simulink model "common_3"  (R2015b)
settings: Solver=ode4  StartTime=0.0  StopTime=tmax  FixedStep=0.001  RelTol=1e-3
undefined symbols (not defined in the file): dq1_init, dq2_init, g, ki, kp, l, l10, l20, para, q1_init, q2_init
settings Model: Creator=Administrator  LastModifiedBy=Administrator

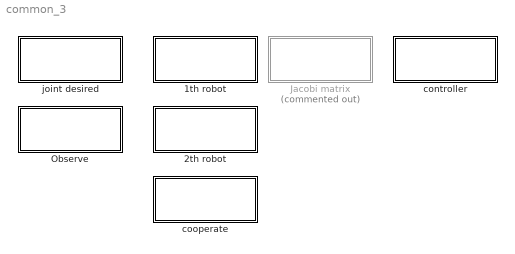
== system common_3 ==
  1th robot : Subsystem
  2th robot : Subsystem
  Jacobi matrix : Subsystem  Commented=on
  Observe : Subsystem
  controller : Subsystem
  cooperate : Subsystem
  joint desired : Subsystem

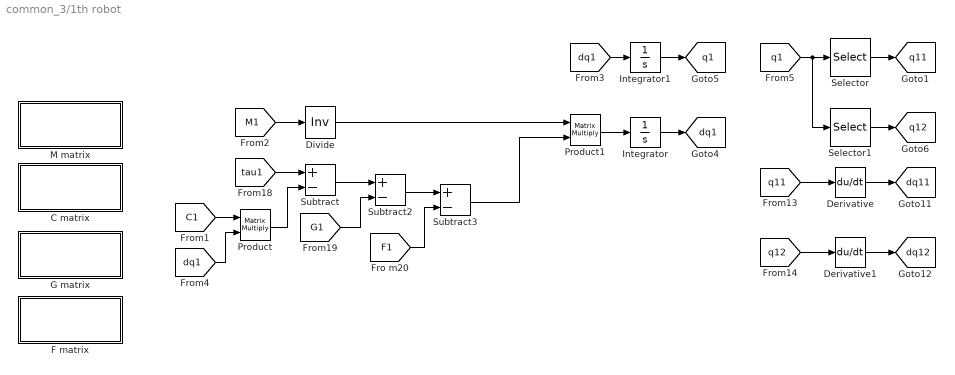
== system common_3/1th robot ==
  C matrix : Subsystem
  Derivative : Derivative
  "Derivative1 " : Derivative
  Divide : Product  Inputs=/  Multiplication=Matrix(*)
  F matrix : Subsystem
  G matrix : Subsystem
  Integrator : Integrator  InitialCondition=dq1_init
  Integrator1 : Integrator  InitialCondition=q1_init
  M matrix : Subsystem
  Product : Product  Multiplication=Matrix(*)
  Product1 : Product  Multiplication=Matrix(*)
  Selector : Selector  InputPortWidth=2  IndexOptions=Index vector (dialog)  Indices=[1]  OutputSizes=1
  Selector1 : Selector  InputPortWidth=2  IndexOptions=Index vector (dialog)  Indices=[2]  OutputSizes=1
  Subtract : Sum  Inputs=+-
  Subtract2 : Sum  Inputs=+-
  Subtract3 : Sum  Inputs=+-
  tag scope: dq11=global, dq12=global, dq1=global, q11=global, q12=global, q1=global
  wires:
  Integrator/1 -> [dq1]
  [dq1] -> Integrator1/1
  Integrator1/1 -> [q1]
  Selector/1 -> [q11]
  Selector1/1 -> [q12]
  [q1] -> Selector/1, Selector1/1
  [q11] -> Derivative/1
  Derivative/1 -> [dq11]
  [q12] -> "Derivative1 "/1
  "Derivative1 "/1 -> [dq12]
  [M1] -> Divide/1
  Product1/1 -> Integrator/1
  Divide/1 -> Product1/1
  [tau1] -> Subtract/1
  [C1] -> Product/1
  Product/1 -> Subtract/2
  Subtract/1 -> Subtract2/1
  [G1] -> Subtract2/2
  Subtract2/1 -> Subtract3/1
  [F1] -> Subtract3/2
  Subtract3/1 -> Product1/2
  [dq1] -> Product/2

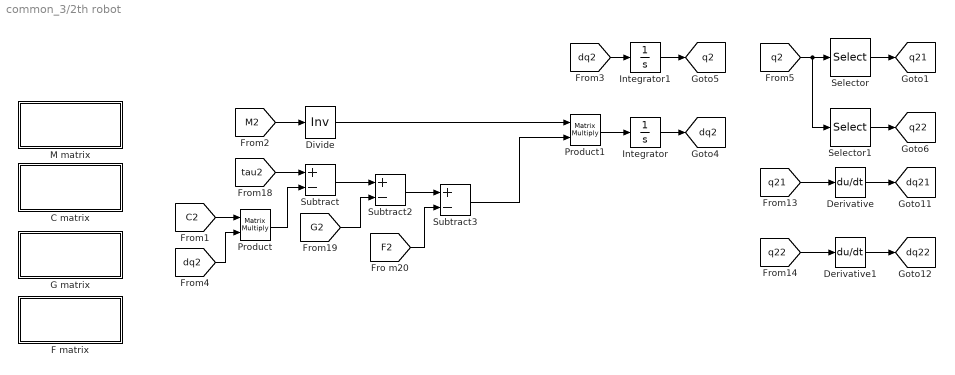
== system common_3/2th robot ==
  C matrix : Subsystem
  Derivative : Derivative
  "Derivative1 " : Derivative
  Divide : Product  Inputs=/  Multiplication=Matrix(*)
  F matrix : Subsystem
  G matrix : Subsystem
  Integrator : Integrator  InitialCondition=dq2_init
  Integrator1 : Integrator  InitialCondition=q2_init
  M matrix : Subsystem
  Product : Product  Multiplication=Matrix(*)
  Product1 : Product  Multiplication=Matrix(*)
  Selector : Selector  InputPortWidth=2  IndexOptions=Index vector (dialog)  Indices=[1]  OutputSizes=1
  Selector1 : Selector  InputPortWidth=2  IndexOptions=Index vector (dialog)  Indices=[2]  OutputSizes=1
  Subtract : Sum  Inputs=+-
  Subtract2 : Sum  Inputs=+-
  Subtract3 : Sum  Inputs=+-
  tag scope: dq21=global, dq22=global, dq2=global, q21=global, q22=global, q2=global
  wires:
  [dq2] -> Product/2
  Subtract3/1 -> Product1/2
  [F2] -> Subtract3/2
  Subtract2/1 -> Subtract3/1
  [G2] -> Subtract2/2
  Subtract/1 -> Subtract2/1
  Product/1 -> Subtract/2
  [C2] -> Product/1
  [tau2] -> Subtract/1
  Divide/1 -> Product1/1
  Product1/1 -> Integrator/1
  [M2] -> Divide/1
  "Derivative1 "/1 -> [dq22]
  [q22] -> "Derivative1 "/1
  Derivative/1 -> [dq21]
  [q21] -> Derivative/1
  [q2] -> Selector1/1, Selector/1
  Selector1/1 -> [q22]
  Selector/1 -> [q21]
  Integrator1/1 -> [q2]
  [dq2] -> Integrator1/1
  Integrator/1 -> [dq2]

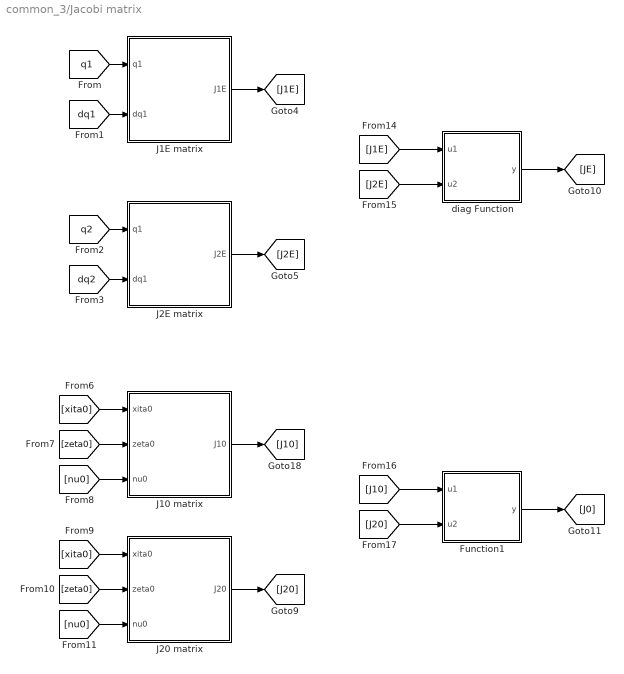
== system common_3/Jacobi matrix ==
  " Function1" : MATLAB Function  TreatAsAtomicUnit=on
  J10 matrix : Subsystem
  J1E matrix : Subsystem
  J20 matrix : Subsystem
  J2E matrix : Subsystem
  diag Function : MATLAB Function  TreatAsAtomicUnit=on
  wires:
  [q1] -> J1E matrix/1(q1)
  [dq1] -> J1E matrix/2(dq1)
  [q2] -> J2E matrix/1(q1)
  [dq2] -> J2E matrix/2(dq1)
  J1E matrix/1(J1E) -> [J1E]
  J2E matrix/1(J2E) -> [J2E]
  [xita0] -> J10 matrix/1(xita0)
  [xita0] -> J20 matrix/1(xita0)
  [zeta0] -> J20 matrix/2(zeta0)
  [nu0] -> J20 matrix/3(nu0)
  [zeta0] -> J10 matrix/2(zeta0)
  [nu0] -> J10 matrix/3(nu0)
  J10 matrix/1(J10) -> [J10]
  J20 matrix/1(J20) -> [J20]
  [J1E] -> diag Function/1(u1)
  [J2E] -> diag Function/2(u2)
  diag Function/1(y) -> [JE]
  [J10] -> " Function1"/1(u1)
  [J20] -> " Function1"/2(u2)
  " Function1"/1(y) -> [J0]

== system common_3/Observe ==
  Scope{,1..4} (5 alike) : Scope  NumInputPorts=4
  wires:
  [q11] -> Scope/1
  [q12] -> Scope/2
  [q21] -> Scope/3
  [q22] -> Scope/4
  [dq11] -> Scope1/1
  [dq12] -> Scope1/2
  [dq21] -> Scope1/3
  [dq22] -> Scope1/4
  [M1] -> Scope2/1
  [C1] -> Scope2/2
  [G1] -> Scope2/3
  [F1] -> Scope2/4
  [M2] -> Scope3/1
  [C2] -> Scope3/2
  [G2] -> Scope3/3
  [F2] -> Scope3/4
  [qd] -> Scope4/1
  [dqd] -> Scope4/2
  [q] -> Scope4/3
  [dq] -> Scope4/4

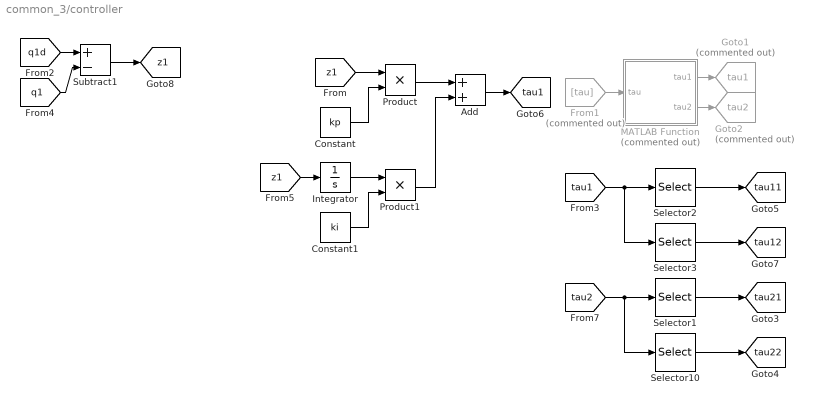
== system common_3/controller ==
  Add : Sum
  Constant : Constant  Value=kp
  Constant1 : Constant  Value=ki
  From1 : From  Commented=on  GotoTag=tau  TagVisibility=global
  Goto1 : Goto  Commented=on  GotoTag=tau1  TagVisibility=global
  Goto2 : Goto  Commented=on  GotoTag=tau2  TagVisibility=global
  Integrator : Integrator
  MATLAB Function : MATLAB Function  Commented=on  TreatAsAtomicUnit=on
  Product : Product
  Product1 : Product
  Selector1 : Selector  InputPortWidth=2  IndexOptions=Index vector (dialog)  Indices=[1]  OutputSizes=1
  Selector10 : Selector  InputPortWidth=2  IndexOptions=Index vector (dialog)  Indices=[2]  OutputSizes=1
  Selector2 : Selector  InputPortWidth=2  IndexOptions=Index vector (dialog)  Indices=[1]  OutputSizes=1
  Selector3 : Selector  InputPortWidth=2  IndexOptions=Index vector (dialog)  Indices=[2]  OutputSizes=1
  Subtract1 : Sum  Inputs=+-
  tag scope: tau11=global, tau12=global, tau1=global, tau21=global, tau22=global, z1=global
  wires:
  [z1] -> Product/1
  Constant/1 -> Product/2
  Product/1 -> Add/1
  Constant1/1 -> Product1/2
  Add/1 -> [tau1]
  From1/1 -> MATLAB Function/1(tau)
  MATLAB Function/1(tau1) -> Goto1/1
  MATLAB Function/2(tau2) -> Goto2/1
  Selector2/1 -> [tau11]
  Selector3/1 -> [tau12]
  [tau1] -> Selector3/1, Selector2/1
  Selector1/1 -> [tau21]
  Selector10/1 -> [tau22]
  [tau2] -> Selector1/1, Selector10/1
  [z1] -> Integrator/1
  Integrator/1 -> Product1/1
  Product1/1 -> Add/2
  [q1d] -> Subtract1/1
  [q1] -> Subtract1/2
  Subtract1/1 -> [z1]

== system common_3/cooperate ==
  MATLAB Function : MATLAB Function  TreatAsAtomicUnit=on
  Matrix Concatenate : Concatenate  Mode=Multidimensional array
  Matrix Concatenate1 : Concatenate  Mode=Multidimensional array
  tag scope: C=global, F=global, G=global, M=global, dq=global, q=global
  wires:
  [M1] -> MATLAB Function/1(M1)
  [M2] -> MATLAB Function/2(M2)
  [C1] -> MATLAB Function/3(C1)
  [C2] -> MATLAB Function/4(C2)
  MATLAB Function/1(M) -> [M]
  MATLAB Function/2(C) -> [C]
  [G1] -> MATLAB Function/5(G1)
  [G2] -> MATLAB Function/6(G2)
  MATLAB Function/3(G) -> [G]
  MATLAB Function/4(F) -> [F]
  [F1] -> MATLAB Function/7(F1)
  [F2] -> MATLAB Function/8(F2)
  [q1] -> Matrix Concatenate/1
  [q2] -> Matrix Concatenate/2
  Matrix Concatenate/1 -> [q]
  [dq1] -> Matrix Concatenate1/1
  [dq2] -> Matrix Concatenate1/2
  Matrix Concatenate1/1 -> [dq]

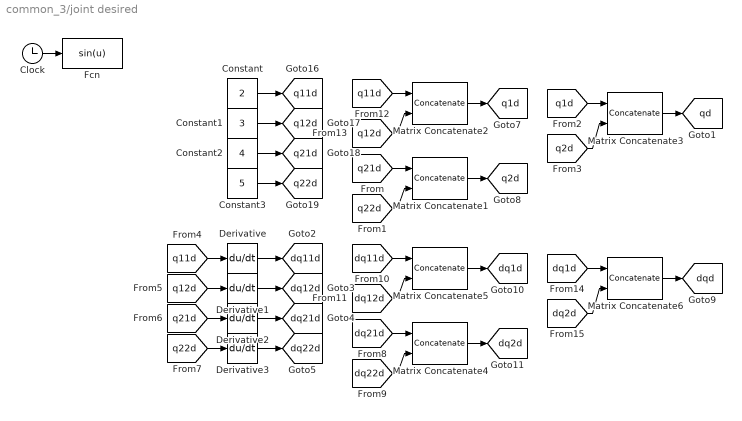
== system common_3/joint desired ==
  Clock : Clock
  Constant : Constant  Value=2
  Constant1 : Constant  Value=3
  Constant2 : Constant  Value=4
  Constant3 : Constant  Value=5
  Derivative{,1..3} (4 alike) : Derivative
  Fcn : Fcn  Expr=sin(u)
  Matrix Concatenate{1..6} (6 alike) : Concatenate  Mode=Multidimensional array
  tag scope: dq11d=global, dq12d=global, dq1d=global, dq21d=global, dq22d=global, dq2d=global, dqd=global, q11d=global, q12d=global, q1d=global, q21d=global, q22d=global, q2d=global, qd=global
  wires:
  Constant/1 -> [q11d]
  Constant3/1 -> [q22d]
  Constant2/1 -> [q21d]
  Constant1/1 -> [q12d]
  [q11d] -> Derivative/1
  Derivative/1 -> [dq11d]
  [q12d] -> Derivative1/1
  Derivative1/1 -> [dq12d]
  [q21d] -> Derivative2/1
  Derivative2/1 -> [dq21d]
  [q22d] -> Derivative3/1
  Derivative3/1 -> [dq22d]
  Matrix Concatenate3/1 -> [qd]
  Clock/1 -> Fcn/1
  [q11d] -> Matrix Concatenate2/1
  [q12d] -> Matrix Concatenate2/2
  Matrix Concatenate2/1 -> [q1d]
  [q21d] -> Matrix Concatenate1/1
  [q22d] -> Matrix Concatenate1/2
  Matrix Concatenate1/1 -> [q2d]
  [q1d] -> Matrix Concatenate3/1
  [q2d] -> Matrix Concatenate3/2
  Matrix Concatenate6/1 -> [dqd]
  [dq11d] -> Matrix Concatenate5/1
  [dq12d] -> Matrix Concatenate5/2
  Matrix Concatenate5/1 -> [dq1d]
  [dq21d] -> Matrix Concatenate4/1
  [dq22d] -> Matrix Concatenate4/2
  Matrix Concatenate4/1 -> [dq2d]
  [dq1d] -> Matrix Concatenate6/1
  [dq2d] -> Matrix Concatenate6/2

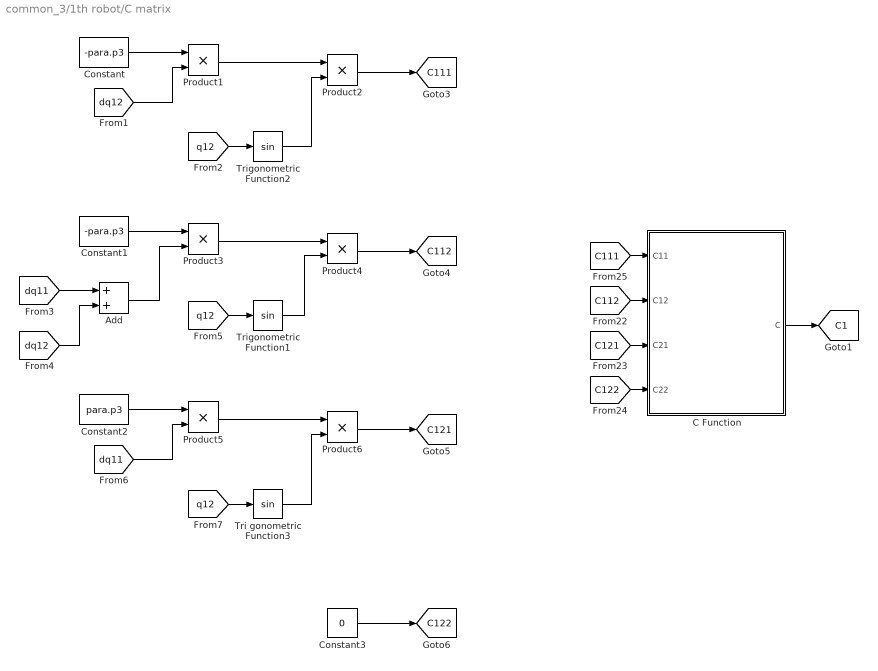
== system common_3/1th robot/C matrix ==
  Add : Sum
  C Function : MATLAB Function  TreatAsAtomicUnit=on
  Constant : Constant  Value=-para.p3
  Constant1 : Constant  Value=-para.p3
  Constant2 : Constant  Value=para.p3
  Constant3 : Constant  Value=0
  Product{1..6} (6 alike) : Product
  Tri gonometric Function3 : Trigonometry
  Trigonometric Function1 : Trigonometry
  Trigonometric Function2 : Trigonometry
  tag scope: C111=global, C112=global, C121=global, C122=global, C1=global
  wires:
  [C111] -> C Function/1(C11)
  [C112] -> C Function/2(C12)
  [C121] -> C Function/3(C21)
  [C122] -> C Function/4(C22)
  Constant/1 -> Product1/1
  [dq12] -> Product1/2
  Product1/1 -> Product2/1
  [q12] -> Trigonometric Function2/1
  Trigonometric Function2/1 -> Product2/2
  Product2/1 -> [C111]
  Constant1/1 -> Product3/1
  [dq11] -> Add/1
  [dq12] -> Add/2
  Add/1 -> Product3/2
  Product3/1 -> Product4/1
  [q12] -> Trigonometric Function1/1
  Trigonometric Function1/1 -> Product4/2
  Product4/1 -> [C112]
  Constant2/1 -> Product5/1
  [dq11] -> Product5/2
  Product5/1 -> Product6/1
  [q12] -> Tri gonometric Function3/1
  Tri gonometric Function3/1 -> Product6/2
  Product6/1 -> [C121]
  Constant3/1 -> [C122]
  C Function/1(C) -> [C1]

== system common_3/1th robot/F matrix ==
  Constant : Constant  Value=0.2
  Constant1 : Constant  Value=0.2
  F Function2 : MATLAB Function  TreatAsAtomicUnit=on
  Product : Product
  Product1 : Product
  Sign : Signum
  Sign1 : Signum
  tag scope: F11=global, F12=global, F1=global
  wires:
  F Function2/1(F) -> [F1]
  [F11] -> F Function2/1(F11)
  [F12] -> F Function2/2(F21)
  Constant/1 -> Product/1
  Sign/1 -> Product/2
  [dq11] -> Sign/1
  Product/1 -> [F11]
  Constant1/1 -> Product1/1
  Sign1/1 -> Product1/2
  [dq12] -> Sign1/1
  Product1/1 -> [F12]

== system common_3/1th robot/G matrix ==
  Constant : Constant  Value=para.p4*g
  Constant1 : Constant  Value=para.p5*g
  Constant2 : Constant  Value=para.p5*g
  G Function1 : MATLAB Function  TreatAsAtomicUnit=on
  Product1 : Product
  Product2 : Product
  Product3 : Product
  Subtract1 : Sum
  Subtract4 : Sum
  Subtract5 : Sum
  Trigonometric Function1 : Trigonometry  Operator=cos
  Trigonometric Function2 : Trigonometry  Operator=cos
  Trigonometric Function3 : Trigonometry  Operator=cos
  tag scope: G11=global, G12=global, G1=global
  wires:
  [G11] -> G Function1/1(G11)
  [G12] -> G Function1/2(G21)
  G Function1/1(G) -> [G1]
  Constant/1 -> Product1/1
  Trigonometric Function2/1 -> Product1/2
  [q11] -> Trigonometric Function2/1
  Product1/1 -> Subtract4/1
  Constant2/1 -> Product2/1
  Subtract5/1 -> Trigonometric Function3/1
  [q11] -> Subtract5/1
  [q12] -> Subtract5/2
  Trigonometric Function3/1 -> Product2/2
  Product2/1 -> Subtract4/2
  Subtract4/1 -> [G11]
  Constant1/1 -> Product3/1
  Subtract1/1 -> Trigonometric Function1/1
  [q11] -> Subtract1/1
  [q12] -> Subtract1/2
  Product3/1 -> [G12]
  Trigonometric Function1/1 -> Product3/2

== system common_3/1th robot/M matrix ==
  Constant1 : Constant  Value=2*para.p3
  Constant2 : Constant  Value=para.p1+para.p2
  Constant3 : Constant  Value=para.p2
  Constant4 : Constant  Value=para.p3
  Constant5 : Constant  Value=para.p2
  M Function1 : MATLAB Function  TreatAsAtomicUnit=on
  Product1 : Product
  Product2 : Product
  Subtract1 : Sum
  Subtract2 : Sum
  Trigonometric Function1 : Trigonometry  Operator=cos
  Trigonometric Function8 : Trigonometry  Operator=cos
  tag scope: M111=global, M112=global, M121=global, M122=global, M1=global
  wires:
  M Function1/1(M) -> [M1]
  [M111] -> M Function1/1(M11)
  [M112] -> M Function1/2(M12)
  [M121] -> M Function1/3(M21)
  [M122] -> M Function1/4(M22)
  [q12] -> Trigonometric Function8/1
  Constant2/1 -> Subtract1/1
  Constant1/1 -> Product1/1
  Trigonometric Function8/1 -> Product1/2
  Product1/1 -> Subtract1/2
  Subtract2/1 -> [M121], [M112]
  Constant5/1 -> [M122]
  Subtract1/1 -> [M111]
  Constant3/1 -> Subtract2/1
  Constant4/1 -> Product2/1
  [q12] -> Trigonometric Function1/1
  Trigonometric Function1/1 -> Product2/2
  Product2/1 -> Subtract2/2

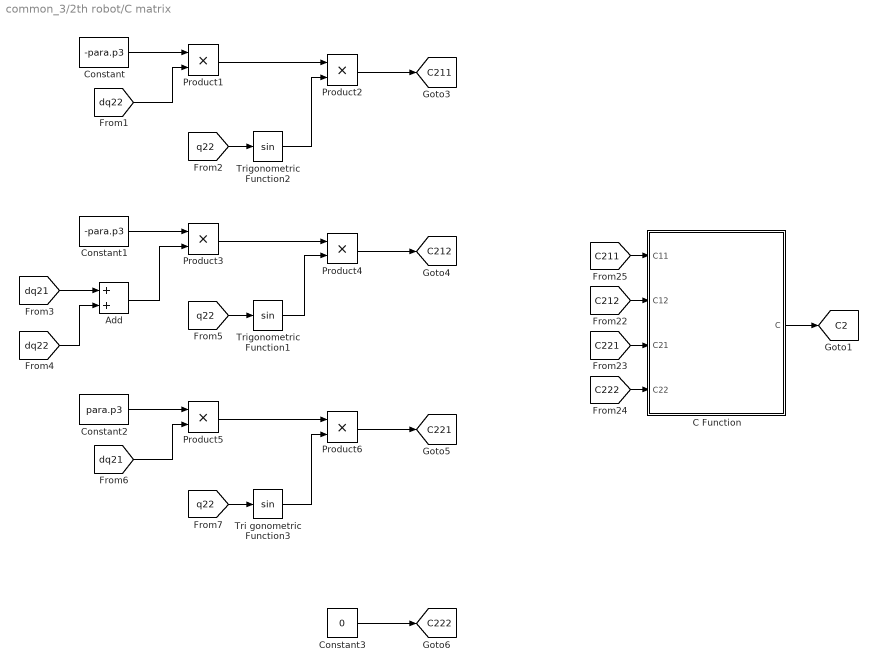
== system common_3/2th robot/C matrix ==
  Add : Sum
  C Function : MATLAB Function  TreatAsAtomicUnit=on
  Constant : Constant  Value=-para.p3
  Constant1 : Constant  Value=-para.p3
  Constant2 : Constant  Value=para.p3
  Constant3 : Constant  Value=0
  Product{1..6} (6 alike) : Product
  Tri gonometric Function3 : Trigonometry
  Trigonometric Function1 : Trigonometry
  Trigonometric Function2 : Trigonometry
  tag scope: C211=global, C212=global, C221=global, C222=global, C2=global
  wires:
  C Function/1(C) -> [C2]
  Constant3/1 -> [C222]
  Product6/1 -> [C221]
  Tri gonometric Function3/1 -> Product6/2
  [q22] -> Tri gonometric Function3/1
  Product5/1 -> Product6/1
  [dq21] -> Product5/2
  Constant2/1 -> Product5/1
  Product4/1 -> [C212]
  Trigonometric Function1/1 -> Product4/2
  [q22] -> Trigonometric Function1/1
  Product3/1 -> Product4/1
  Add/1 -> Product3/2
  [dq22] -> Add/2
  [dq21] -> Add/1
  Constant1/1 -> Product3/1
  Product2/1 -> [C211]
  Trigonometric Function2/1 -> Product2/2
  [q22] -> Trigonometric Function2/1
  Product1/1 -> Product2/1
  [dq22] -> Product1/2
  Constant/1 -> Product1/1
  [C222] -> C Function/4(C22)
  [C221] -> C Function/3(C21)
  [C212] -> C Function/2(C12)
  [C211] -> C Function/1(C11)

== system common_3/2th robot/F matrix ==
  Constant : Constant  Value=0.2
  Constant1 : Constant  Value=0.2
  F Function2 : MATLAB Function  TreatAsAtomicUnit=on
  Product : Product
  Product1 : Product
  Sign : Signum
  Sign1 : Signum
  tag scope: F21=global, F22=global, F2=global
  wires:
  Product1/1 -> [F22]
  [dq22] -> Sign1/1
  Sign1/1 -> Product1/2
  Constant1/1 -> Product1/1
  Product/1 -> [F21]
  [dq21] -> Sign/1
  Sign/1 -> Product/2
  Constant/1 -> Product/1
  [F22] -> F Function2/2(F21)
  [F21] -> F Function2/1(F11)
  F Function2/1(F) -> [F2]

== system common_3/2th robot/G matrix ==
  Constant : Constant  Value=para.p4*g
  Constant1 : Constant  Value=para.p5*g
  Constant2 : Constant  Value=para.p5*g
  G Function1 : MATLAB Function  TreatAsAtomicUnit=on
  Product1 : Product
  Product2 : Product
  Product3 : Product
  Subtract1 : Sum
  Subtract4 : Sum
  Subtract5 : Sum
  Trigonometric Function1 : Trigonometry  Operator=cos
  Trigonometric Function2 : Trigonometry  Operator=cos
  Trigonometric Function3 : Trigonometry  Operator=cos
  tag scope: G21=global, G22=global, G2=global
  wires:
  Trigonometric Function1/1 -> Product3/2
  Product3/1 -> [G22]
  [q22] -> Subtract1/2
  [q21] -> Subtract1/1
  Subtract1/1 -> Trigonometric Function1/1
  Constant1/1 -> Product3/1
  Subtract4/1 -> [G21]
  Product2/1 -> Subtract4/2
  Trigonometric Function3/1 -> Product2/2
  [q22] -> Subtract5/2
  [q21] -> Subtract5/1
  Subtract5/1 -> Trigonometric Function3/1
  Constant2/1 -> Product2/1
  Product1/1 -> Subtract4/1
  [q21] -> Trigonometric Function2/1
  Trigonometric Function2/1 -> Product1/2
  Constant/1 -> Product1/1
  G Function1/1(G) -> [G2]
  [G22] -> G Function1/2(G21)
  [G21] -> G Function1/1(G11)

== system common_3/2th robot/M matrix ==
  Constant1 : Constant  Value=2*para.p3
  Constant2 : Constant  Value=para.p1+para.p2
  Constant3 : Constant  Value=para.p2
  Constant4 : Constant  Value=para.p3
  Constant5 : Constant  Value=para.p2
  M Function1 : MATLAB Function  TreatAsAtomicUnit=on
  Product1 : Product
  Product2 : Product
  Subtract1 : Sum
  Subtract2 : Sum
  Trigonometric Function1 : Trigonometry  Operator=cos
  Trigonometric Function8 : Trigonometry  Operator=cos
  tag scope: M211=global, M212=global, M221=global, M222=global, M2=global
  wires:
  Product2/1 -> Subtract2/2
  Trigonometric Function1/1 -> Product2/2
  [q22] -> Trigonometric Function1/1
  Constant4/1 -> Product2/1
  Constant3/1 -> Subtract2/1
  Subtract1/1 -> [M211]
  Constant5/1 -> [M222]
  Subtract2/1 -> [M212], [M221]
  Product1/1 -> Subtract1/2
  Trigonometric Function8/1 -> Product1/2
  Constant1/1 -> Product1/1
  Constant2/1 -> Subtract1/1
  [q22] -> Trigonometric Function8/1
  [M222] -> M Function1/4(M22)
  [M221] -> M Function1/3(M21)
  [M212] -> M Function1/2(M12)
  [M211] -> M Function1/1(M11)
  M Function1/1(M) -> [M2]

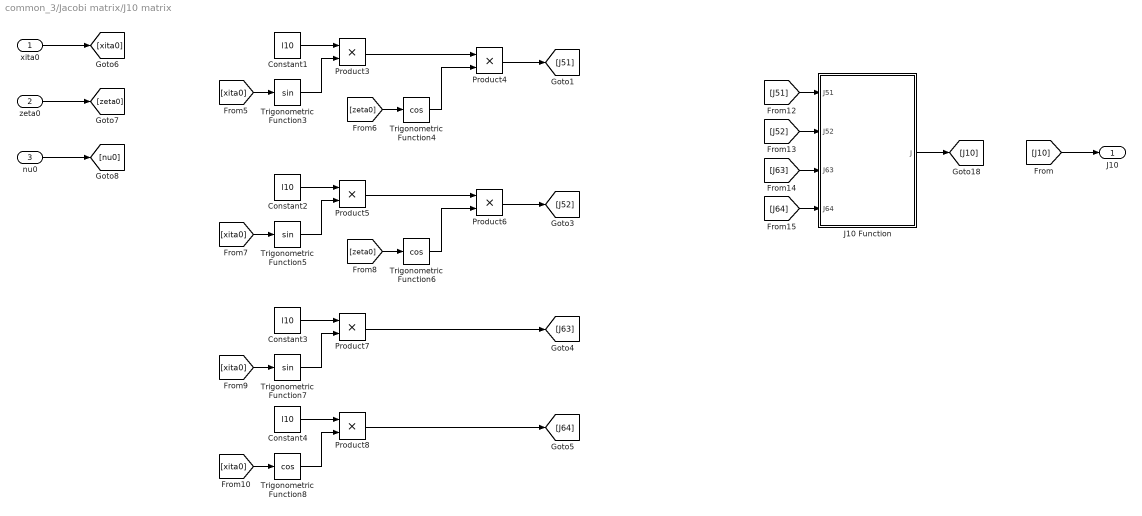
== system common_3/Jacobi matrix/J10 matrix ==
  xita0 : Inport
  zeta0 : Inport  Port=2
  nu0 : Inport  Port=3
  Constant{1..4} (4 alike) : Constant  Value=l10
  J10 Function : MATLAB Function  TreatAsAtomicUnit=on
  Product{3..8} (6 alike) : Product
  Trigonometric Function3 : Trigonometry
  Trigonometric Function4 : Trigonometry  Operator=cos
  Trigonometric Function5 : Trigonometry
  Trigonometric Function6 : Trigonometry  Operator=cos
  Trigonometric Function7 : Trigonometry
  Trigonometric Function8 : Trigonometry  Operator=cos
  J10 : Outport
  wires:
  J10 Function/1(J) -> [J10]
  [J10] -> J10/1
  xita0/1 -> [xita0]
  zeta0/1 -> [zeta0]
  nu0/1 -> [nu0]
  Constant1/1 -> Product3/1
  Product3/1 -> Product4/1
  [xita0] -> Trigonometric Function3/1
  Trigonometric Function3/1 -> Product3/2
  [zeta0] -> Trigonometric Function4/1
  Trigonometric Function4/1 -> Product4/2
  Product4/1 -> [J51]
  Constant2/1 -> Product5/1
  Product5/1 -> Product6/1
  [xita0] -> Trigonometric Function5/1
  Trigonometric Function5/1 -> Product5/2
  [zeta0] -> Trigonometric Function6/1
  Trigonometric Function6/1 -> Product6/2
  Product6/1 -> [J52]
  [xita0] -> Trigonometric Function7/1
  Trigonometric Function7/1 -> Product7/2
  Product7/1 -> [J63]
  Constant3/1 -> Product7/1
  [xita0] -> Trigonometric Function8/1
  Trigonometric Function8/1 -> Product8/2
  Product8/1 -> [J64]
  Constant4/1 -> Product8/1
  [J52] -> J10 Function/2(J52)
  [J63] -> J10 Function/3(J63)
  [J64] -> J10 Function/4(J64)
  [J51] -> J10 Function/1(J51)

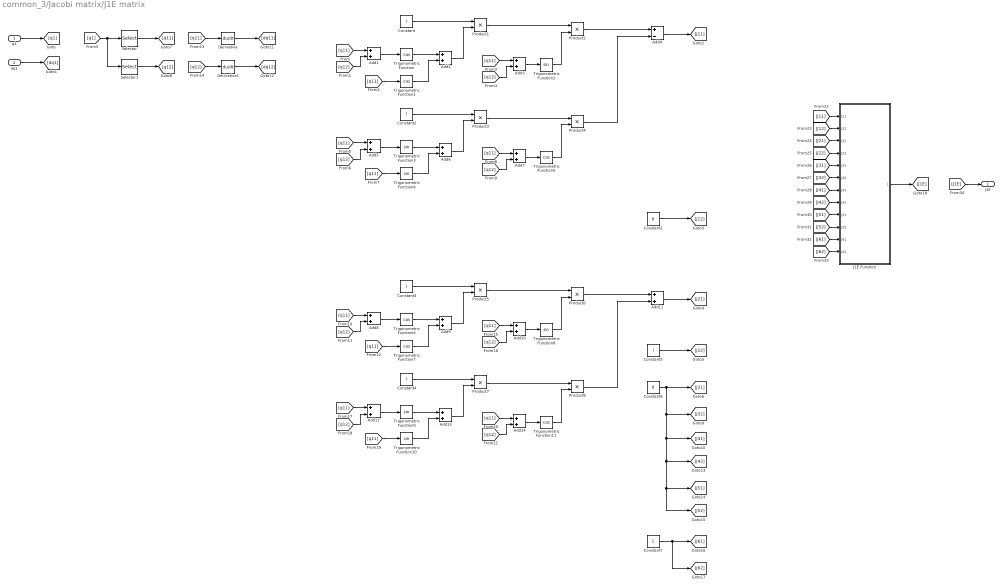
== system common_3/Jacobi matrix/J1E matrix ==
  q1 : Inport
  dq1 : Inport  Port=2
  Add{1..3,5..14} (13 alike) : Sum
  Add4 : Sum  Inputs=+-
  Constant{,2..5} (5 alike) : Constant  Value=l
  Constant1 : Constant  Value=0
  Constant6 : Constant  Value=0
  Constant7 : Constant
  Derivative : Derivative
  Derivative1 : Derivative
  J1E Function : MATLAB Function  TreatAsAtomicUnit=on
  Product{1..8} (8 alike) : Product
  Selector : Selector  InputPortWidth=2  IndexOptions=Index vector (dialog)  Indices=[1]  OutputSizes=1
  Selector1 : Selector  InputPortWidth=2  IndexOptions=Index vector (dialog)  Indices=[2]  OutputSizes=1
  Trigonometric Function{,1,5..7,11} (6 alike) : Trigonometry  Operator=cos
  Trigonometric Function{2..4,8..10} (6 alike) : Trigonometry
  J1E : Outport
  wires:
  q1/1 -> [q1]
  dq1/1 -> [dq1]
  Selector/1 -> [q11]
  Selector1/1 -> [q12]
  [q1] -> Selector1/1, Selector/1
  [q11] -> Derivative/1
  Derivative/1 -> [dq11]
  [q12] -> Derivative1/1
  Derivative1/1 -> [dq12]
  Constant/1 -> Product1/1
  [q11] -> Add1/1
  [q12] -> Add1/2
  Add1/1 -> Trigonometric Function/1
  Trigonometric Function/1 -> Add2/1
  [q11] -> Trigonometric Function1/1
  Trigonometric Function1/1 -> Add2/2
  Add2/1 -> Product1/2
  Product1/1 -> Product2/1
  [q11] -> Add3/1
  [q12] -> Add3/2
  Add3/1 -> Trigonometric Function2/1
  Trigonometric Function2/1 -> Product2/2
  Constant1/1 -> [J12]
  Product2/1 -> Add4/1
  Constant2/1 -> Product3/1
  [q11] -> Add5/1
  [q12] -> Add5/2
  Add5/1 -> Trigonometric Function3/1
  Trigonometric Function3/1 -> Add6/1
  [q11] -> Trigonometric Function4/1
  Trigonometric Function4/1 -> Add6/2
  Add6/1 -> Product3/2
  Product3/1 -> Product4/1
  [q11] -> Add7/1
  [q12] -> Add7/2
  Add7/1 -> Trigonometric Function5/1
  Trigonometric Function5/1 -> Product4/2
  Product4/1 -> Add4/2
  Add4/1 -> [J11]
  Constant3/1 -> Product5/1
  [q11] -> Add8/1
  [q12] -> Add8/2
  Add8/1 -> Trigonometric Function6/1
  Trigonometric Function6/1 -> Add9/1
  [q11] -> Trigonometric Function7/1
  Trigonometric Function7/1 -> Add9/2
  Add9/1 -> Product5/2
  Product5/1 -> Product6/1
  [q11] -> Add10/1
  [q12] -> Add10/2
  Add10/1 -> Trigonometric Function8/1
  Trigonometric Function8/1 -> Product6/2
  Product6/1 -> Add11/1
  Constant4/1 -> Product7/1
  [q11] -> Add12/1
  [q12] -> Add12/2
  Add12/1 -> Trigonometric Function9/1
  Trigonometric Function9/1 -> Add13/1
  [q11] -> Trigonometric Function10/1
  Trigonometric Function10/1 -> Add13/2
  Add13/1 -> Product7/2
  Product7/1 -> Product8/1
  [q11] -> Add14/1
  [q12] -> Add14/2
  Add14/1 -> Trigonometric Function11/1
  Trigonometric Function11/1 -> Product8/2
  Product8/1 -> Add11/2
  Add11/1 -> [J21]
  Constant5/1 -> [J22]
  Constant6/1 -> [J32], [J41], [J42], [J51], [J52], [J31]
  Constant7/1 -> [J62], [J61]
  [J12] -> J1E Function/2(J12)
  [J32] -> J1E Function/6(J32)
  [J11] -> J1E Function/1(J11)
  [J21] -> J1E Function/3(J21)
  [J22] -> J1E Function/4(J22)
  [J31] -> J1E Function/5(J31)
  [J41] -> J1E Function/7(J41)
  [J42] -> J1E Function/8(J42)
  [J51] -> J1E Function/9(J51)
  [J52] -> J1E Function/10(J52)
  [J61] -> J1E Function/11(J61)
  [J62] -> J1E Function/12(J62)
  J1E Function/1(J) -> [J1E]
  [J1E] -> J1E/1

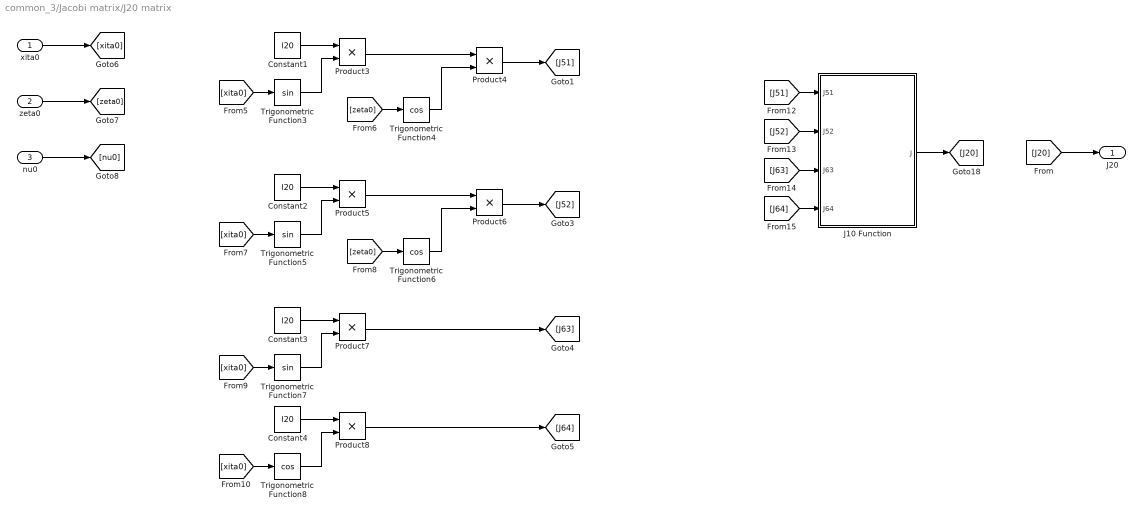
== system common_3/Jacobi matrix/J20 matrix ==
  xita0 : Inport
  zeta0 : Inport  Port=2
  nu0 : Inport  Port=3
  Constant{1..4} (4 alike) : Constant  Value=l20
  J10 Function : MATLAB Function  TreatAsAtomicUnit=on
  Product{3..8} (6 alike) : Product
  Trigonometric Function3 : Trigonometry
  Trigonometric Function4 : Trigonometry  Operator=cos
  Trigonometric Function5 : Trigonometry
  Trigonometric Function6 : Trigonometry  Operator=cos
  Trigonometric Function7 : Trigonometry
  Trigonometric Function8 : Trigonometry  Operator=cos
  J20 : Outport
  wires:
  [J51] -> J10 Function/1(J51)
  [J64] -> J10 Function/4(J64)
  [J63] -> J10 Function/3(J63)
  [J52] -> J10 Function/2(J52)
  Constant4/1 -> Product8/1
  Product8/1 -> [J64]
  Trigonometric Function8/1 -> Product8/2
  [xita0] -> Trigonometric Function8/1
  Constant3/1 -> Product7/1
  Product7/1 -> [J63]
  Trigonometric Function7/1 -> Product7/2
  [xita0] -> Trigonometric Function7/1
  Product6/1 -> [J52]
  Trigonometric Function6/1 -> Product6/2
  [zeta0] -> Trigonometric Function6/1
  Trigonometric Function5/1 -> Product5/2
  [xita0] -> Trigonometric Function5/1
  Product5/1 -> Product6/1
  Constant2/1 -> Product5/1
  Product4/1 -> [J51]
  Trigonometric Function4/1 -> Product4/2
  [zeta0] -> Trigonometric Function4/1
  Trigonometric Function3/1 -> Product3/2
  [xita0] -> Trigonometric Function3/1
  Product3/1 -> Product4/1
  Constant1/1 -> Product3/1
  nu0/1 -> [nu0]
  zeta0/1 -> [zeta0]
  xita0/1 -> [xita0]
  [J20] -> J20/1
  J10 Function/1(J) -> [J20]

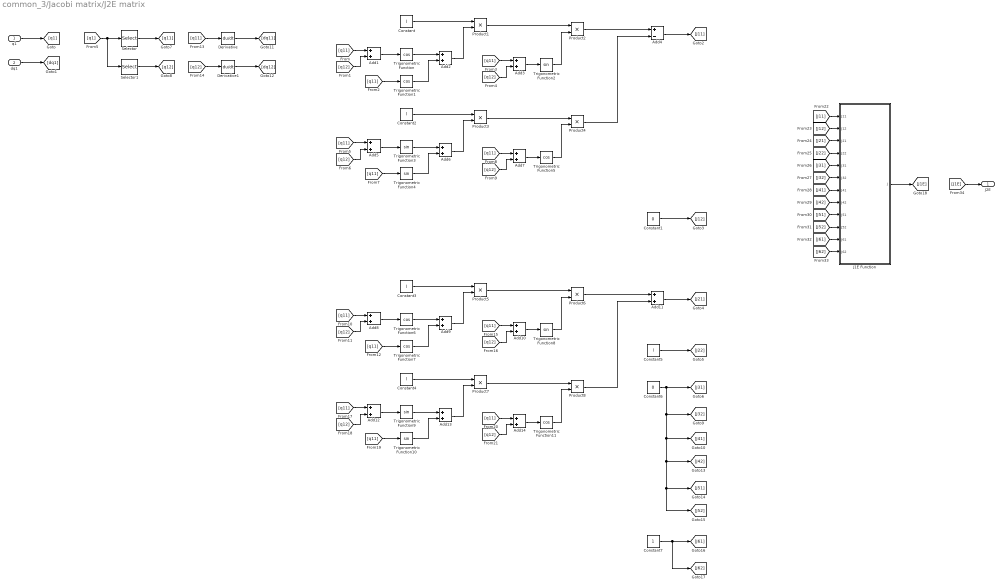
== system common_3/Jacobi matrix/J2E matrix ==
  q1 : Inport
  dq1 : Inport  Port=2
  Add{1..3,5..14} (13 alike) : Sum
  Add4 : Sum  Inputs=+-
  Constant{,2..5} (5 alike) : Constant  Value=l
  Constant1 : Constant  Value=0
  Constant6 : Constant  Value=0
  Constant7 : Constant
  Derivative : Derivative
  Derivative1 : Derivative
  J1E Function : MATLAB Function  TreatAsAtomicUnit=on
  Product{1..8} (8 alike) : Product
  Selector : Selector  InputPortWidth=2  IndexOptions=Index vector (dialog)  Indices=[1]  OutputSizes=1
  Selector1 : Selector  InputPortWidth=2  IndexOptions=Index vector (dialog)  Indices=[2]  OutputSizes=1
  Trigonometric Function{,1,5..7,11} (6 alike) : Trigonometry  Operator=cos
  Trigonometric Function{2..4,8..10} (6 alike) : Trigonometry
  J2E : Outport
  wires:
  [J1E] -> J2E/1
  J1E Function/1(J) -> [J1E]
  [J62] -> J1E Function/12(J62)
  [J61] -> J1E Function/11(J61)
  [J52] -> J1E Function/10(J52)
  [J51] -> J1E Function/9(J51)
  [J42] -> J1E Function/8(J42)
  [J41] -> J1E Function/7(J41)
  [J31] -> J1E Function/5(J31)
  [J22] -> J1E Function/4(J22)
  [J21] -> J1E Function/3(J21)
  [J11] -> J1E Function/1(J11)
  [J32] -> J1E Function/6(J32)
  [J12] -> J1E Function/2(J12)
  Constant7/1 -> [J61], [J62]
  Constant6/1 -> [J31], [J52], [J51], [J42], [J41], [J32]
  Constant5/1 -> [J22]
  Add11/1 -> [J21]
  Product8/1 -> Add11/2
  Trigonometric Function11/1 -> Product8/2
  Add14/1 -> Trigonometric Function11/1
  [q12] -> Add14/2
  [q11] -> Add14/1
  Product7/1 -> Product8/1
  Add13/1 -> Product7/2
  Trigonometric Function10/1 -> Add13/2
  [q11] -> Trigonometric Function10/1
  Trigonometric Function9/1 -> Add13/1
  Add12/1 -> Trigonometric Function9/1
  [q12] -> Add12/2
  [q11] -> Add12/1
  Constant4/1 -> Product7/1
  Product6/1 -> Add11/1
  Trigonometric Function8/1 -> Product6/2
  Add10/1 -> Trigonometric Function8/1
  [q12] -> Add10/2
  [q11] -> Add10/1
  Product5/1 -> Product6/1
  Add9/1 -> Product5/2
  Trigonometric Function7/1 -> Add9/2
  [q11] -> Trigonometric Function7/1
  Trigonometric Function6/1 -> Add9/1
  Add8/1 -> Trigonometric Function6/1
  [q12] -> Add8/2
  [q11] -> Add8/1
  Constant3/1 -> Product5/1
  Add4/1 -> [J11]
  Product4/1 -> Add4/2
  Trigonometric Function5/1 -> Product4/2
  Add7/1 -> Trigonometric Function5/1
  [q12] -> Add7/2
  [q11] -> Add7/1
  Product3/1 -> Product4/1
  Add6/1 -> Product3/2
  Trigonometric Function4/1 -> Add6/2
  [q11] -> Trigonometric Function4/1
  Trigonometric Function3/1 -> Add6/1
  Add5/1 -> Trigonometric Function3/1
  [q12] -> Add5/2
  [q11] -> Add5/1
  Constant2/1 -> Product3/1
  Product2/1 -> Add4/1
  Constant1/1 -> [J12]
  Trigonometric Function2/1 -> Product2/2
  Add3/1 -> Trigonometric Function2/1
  [q12] -> Add3/2
  [q11] -> Add3/1
  Product1/1 -> Product2/1
  Add2/1 -> Product1/2
  Trigonometric Function1/1 -> Add2/2
  [q11] -> Trigonometric Function1/1
  Trigonometric Function/1 -> Add2/1
  Add1/1 -> Trigonometric Function/1
  [q12] -> Add1/2
  [q11] -> Add1/1
  Constant/1 -> Product1/1
  Derivative1/1 -> [dq12]
  [q12] -> Derivative1/1
  Derivative/1 -> [dq11]
  [q11] -> Derivative/1
  [q1] -> Selector/1, Selector1/1
  Selector1/1 -> [q12]
  Selector/1 -> [q11]
  dq1/1 -> [dq1]
  q1/1 -> [q1]

== matlab function common_3/Jacobi matrix/diag Function ==
  data: u1 input; y output; u2 input
function y = fcn(u1,u2)
%#codegen

y = blkdiag(u1,u2);

== matlab function common_3/1th robot/F matrix/F Function2 ==
  data: F11 input; F output; F21 input
function F = fcn(F11,F21)
%#codegen

F = [F11;F21];

== matlab function common_3/1th robot/C matrix/C Function ==
  data: C11 input; C output; C12 input; C21 input; C22 input
function C = fcn(C11,C12,C21,C22)
%#codegen

C = [C11 C12;C21 C22];

== matlab function common_3/1th robot/G matrix/G Function1 ==
  data: G11 input; G output; G21 input
function G = fcn(G11,G21)
%#codegen

G = [G11;G21];

== matlab function common_3/controller/MATLAB Function ==
  data: tau input; tau1 output; tau2 output
function [tau1,tau2]= fcn(tau)
%#codegen

tau1=[tau(1);tau(2)];
tau2=[tau(3);tau(4)];

== matlab function common_3/Jacobi matrix/J1E matrix/J1E Function ==
  data: J11 input; J output; J12 input; J21 input; J22 input; J31 input; J32 input; J41 input; J42 input; J51 input; J52 input; J61 input; J62 input
function J = fcn(J11,J12,J21,J22,J31,J32,J41,J42,J51,J52,J61,J62)
%#codegen

J = [J11 J12;
     J21 J22;
     J31 J32;
     J41 J42;
     J51 J52;
     J61 J62];

== matlab function common_3/Jacobi matrix/J2E matrix/J1E Function ==
  data: J11 input; J output; J12 input; J21 input; J22 input; J31 input; J32 input; J41 input; J42 input; J51 input; J52 input; J61 input; J62 input
function J = fcn(J11,J12,J21,J22,J31,J32,J41,J42,J51,J52,J61,J62)
%#codegen

J = [J11 J12;
     J21 J22;
     J31 J32;
     J41 J42;
     J51 J52;
     J61 J62];

== matlab function common_3/Jacobi matrix/J10 matrix/J10 Function ==
  data: J51 input; J52 input; J output; J63 input; J64 input
function J = fcn(J51,J52,J63,J64)
%#codegen

J = [1 0 0 0 0 0;
     0 1 0 0 0 0;
     0 0 1 0 0 0;
     0 0 0 1 0 0;
     J51 J52 0 0 1 0;
     0 0 J63 J64 0 1;];

== matlab function common_3/Jacobi matrix/J20 matrix/J10 Function ==
  data: J51 input; J52 input; J output; J63 input; J64 input
function J = fcn(J51,J52,J63,J64)
%#codegen

J = [1 0 0 0 0 0;
     0 1 0 0 0 0;
     0 0 1 0 0 0;
     0 0 0 1 0 0;
     J51 J52 0 0 1 0;
     0 0 J63 J64 0 1;];

== matlab function common_3/Jacobi matrix/ Function1 ==
  data: u1 input; y output; u2 input
function y = fcn(u1,u2)
%#codegen

y = [u1';u2'];

== matlab function common_3/1th robot/M matrix/M Function1 ==
  data: M11 input; M output; M12 input; M21 input; M22 input
function M = fcn(M11,M12,M21,M22)
%#codegen

M = [M11 M12;M21 M22];

== matlab function common_3/2th robot/C matrix/C Function ==
  data: C11 input; C output; C12 input; C21 input; C22 input
function C = fcn(C11,C12,C21,C22)
%#codegen

C = [C11 C12;C21 C22];

== matlab function common_3/2th robot/F matrix/F Function2 ==
  data: F11 input; F output; F21 input
function F = fcn(F11,F21)
%#codegen

F = [F11;F21];

== matlab function common_3/2th robot/G matrix/G Function1 ==
  data: G11 input; G output; G21 input
function G = fcn(G11,G21)
%#codegen

G = [G11;G21];

== matlab function common_3/2th robot/M matrix/M Function1 ==
  data: M11 input; M output; M12 input; M21 input; M22 input
function M = fcn(M11,M12,M21,M22)
%#codegen

M = [M11 M12;M21 M22];

== matlab function common_3/cooperate/MATLAB Function ==
  data: M1 input; M output; M2 input; C1 input; C2 input; C output; G1 input; G2 input; G output; F1 input; F2 input; F output
function [M,C,G,F]= fcn(M1,M2,C1,C2,G1,G2,F1,F2)
%#codegen

M=blkdiag(M1,M2);
C=blkdiag(C1,C2);
G=[G1;G2];
F=[F1;F2];
